simulink model "model_identification"  (R2016b)
settings: Solver=ode45  StartTime=0.0  StopTime=T  RelTol=1e-3  EnableMultiTasking=on
model workspace: external: MATLAB File /Users/Ortix/Documents/MATLAB/control-system-lab/nick/matlab/params.m (data not in the file)
values from neighbouring files (symbols this model uses):
  h = 0.01    [par_struct.m]    (also in parameters.m)
  k_m = 50    [getLinearModel.m]    (also in par_struct.m; parameters.m = 41.0587)
  tau_e = 0.03    [getLinearModel.m]    (also in par_struct.m; parameters.m = 0.0312)
settings Model: Creator=Nathan  LastModifiedBy=Ortix
settings DataIOCC: InitialState=states  LimitDataPoints=on  SaveFormat=Array
settings OptimizationCC: LifeSpan=inf
settings DebuggingCC: AllowSymbolicDim=off  SFUnexpectedBacktrackingDiag=warning  SFNoUnconditionalDefaultTransitionDiag=warning  SFExecutionAtInitializationDiag=none
settings HardwareCC: ProdBitPerPointer=32  ProdBitPerSizeT=32  ProdBitPerPtrDiffT=32  ProdLargestAtomicFloat=None  ProdIntDivRoundTo=Undefined  ProdEndianess=Unspecified  ProdWordSize=32  ProdHWDeviceType=32-bit Generic
settings ModelReferenceCC: PropagateSignalLabelsOutOfModel=off
settings GRTTargetCC: TargetLangStandard=C89/C90 (ANSI)  GeneratePreprocessorConditionals=Disable all
settings ConfigComp: CovMetricSettings=dw  CovHtmlReporting=on  CovSaveCumulativeToWorkspaceVar=on  CovSaveSingleToWorkspaceVar=on  CovExternalEMLEnable=off

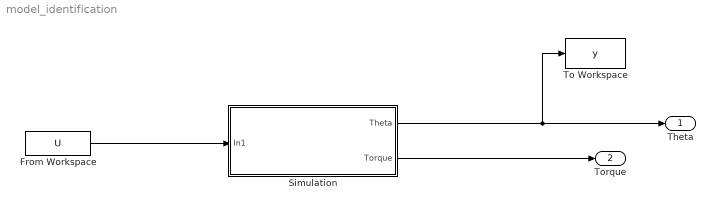
== system model_identification ==
  From Workspace : FromWorkspace  VariableName=U  SampleTime=0
  "Simulation " : Subsystem
  To Workspace : ToWorkspace  VariableName=y  SampleTime=h
  Theta : Outport
  Torque : Outport  Port=2
  wires:
  From Workspace/1 -> "Simulation "/1(In1)
  "Simulation "/2(Torque) -> Torque/1
  "Simulation "/1(Theta) -> To Workspace/1, Theta/1

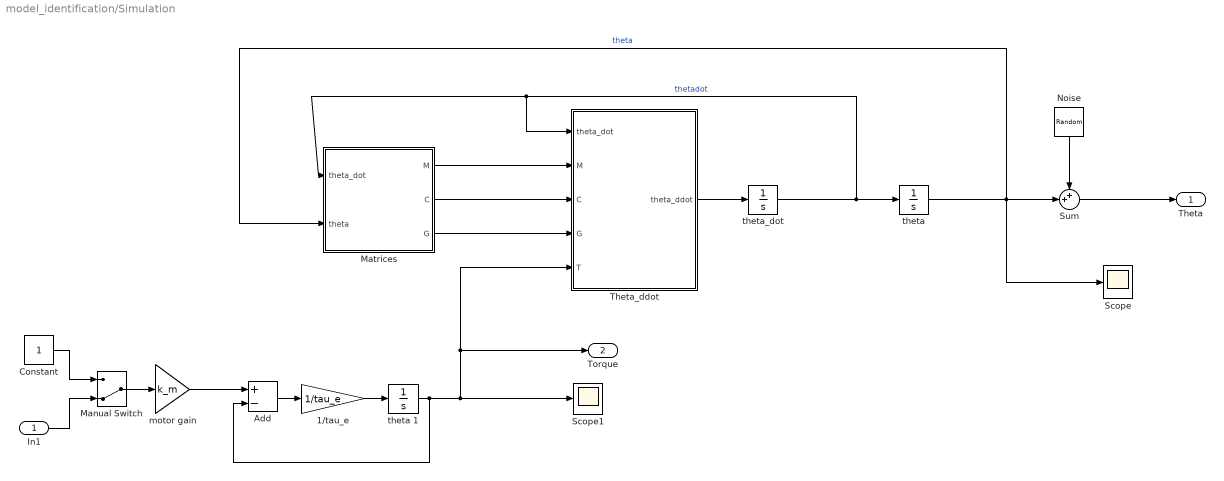
== system model_identification/Simulation  ==
  In1 : Inport
  "1/tau_e " : Gain  Gain=1/tau_e
  Add : Sum  Inputs=+-
  Constant : Constant
  Manual Switch : ManualSwitch  CurrentSetting=0
  Matrices : MATLAB Function  TreatAsAtomicUnit=on
  Noise : RandomNumber  Variance=1e-7  SampleTime=h
  Scope : Scope
  Scope1 : Scope
  Sum : Sum  Inputs=++|
  "Theta_ddot " : MATLAB Function  TreatAsAtomicUnit=on
  "motor gain " : Gain  Gain=k_m
  "theta " : Integrator
  theta 1 : Integrator
  "theta_dot " : Integrator
  Theta : Outport
  Torque : Outport  Port=2
  wires:
  Manual Switch/1 -> "motor gain "/1
  theta 1/1 -> Add/2, Torque/1, "Theta_ddot "/5(T), Scope1/1
  "theta_dot "/1 -> "theta "/1, "Theta_ddot "/1(theta_dot), Matrices/1(theta_dot)  "thetadot"
  Matrices/3(G) -> "Theta_ddot "/4(G)
  In1/1 -> Manual Switch/2
  Constant/1 -> Manual Switch/1
  Noise/1 -> Sum/1
  Matrices/1(M) -> "Theta_ddot "/2(M)
  "motor gain "/1 -> Add/1
  "Theta_ddot "/1(theta_ddot) -> "theta_dot "/1
  Matrices/2(C) -> "Theta_ddot "/3(C)
  Add/1 -> "1/tau_e "/1
  "1/tau_e "/1 -> theta 1/1
  Sum/1 -> Theta/1
  "theta "/1 -> Sum/2, Scope/1, Matrices/2(theta)  "theta"

== matlab function model_identification/Simulation /Theta_ddot  ==
  data: theta_dot input; M input; C input; G input; theta_ddot output; T input
function theta_ddot = fcn(theta_dot,M,C,G,T)
theta_ddot = [0;0];

theta_ddot = M\[T;0] - M\C*theta_dot - M\G;

== matlab function model_identification/Simulation /Matrices ==
  data: theta_dot input; theta input; M output; C output; G output
function [M, C, G] = fcn(theta_dot, theta)

M = zeros(2);
C = zeros(2);
G = [0;0];

g = 9.81; 
l1 = 0.1;
l2 = 0.1;
m1 = 0.125;
m2 = 0.05;
c1 = 0.04; % Keeping it negative results in no motion at all, -0.04 or + 0.04?
c2 = 0.06;
I1 = 0.074;
I2 = 0.00012;
b1 = 4.8;
b2 = 0.0002;

P1 = m1*c1^2+m2*l1^2+I1;
P2 = m2*c2^2+ I2;
P3 = m2*l1*c2;
g1 = (m1*c1+m2*l1)*g;
g2 = m2*c2*g;

M = [(P1 + P2 + 2*P3*cos(theta(2)))               (P2 + P3*cos(theta(2))) ;
     (P2 + P3*cos(theta(2)))                       P2                   ];
 
 
C = [(b1 - P3*theta_dot(2)*sin(theta(2)))           (-P3*(theta_dot(1)+theta_dot(2))*sin(theta(2))) ;
     (P3*theta_dot(1)*sin(theta(2)))                 b2                                      ];
     
G = [(-g1*sin(theta(1))-g2*sin(theta(1) + theta(2))) ;
      -g2*sin(theta(1)+theta(2))                   ];
